simulink model "fuzzy_AG"  (R2022b)
settings: Solver=VariableStepAuto  StartTime=0.0  StopTime=20000  RelTol=1e-3
libraries: fuzblock x1
settings Model: Creator=Juan Jose Restrepo  LastModifiedBy=mluser

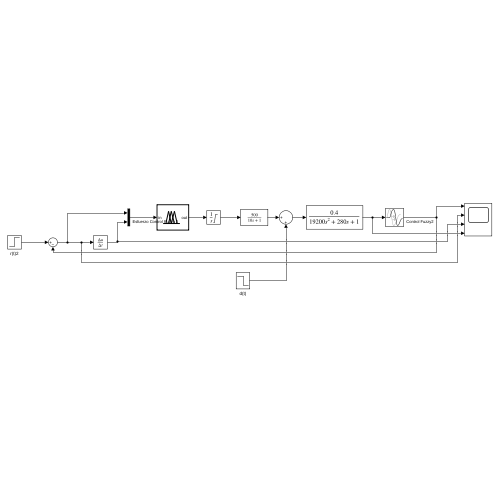
[thumbnail: Simulink's stored preview of the top-level diagram]
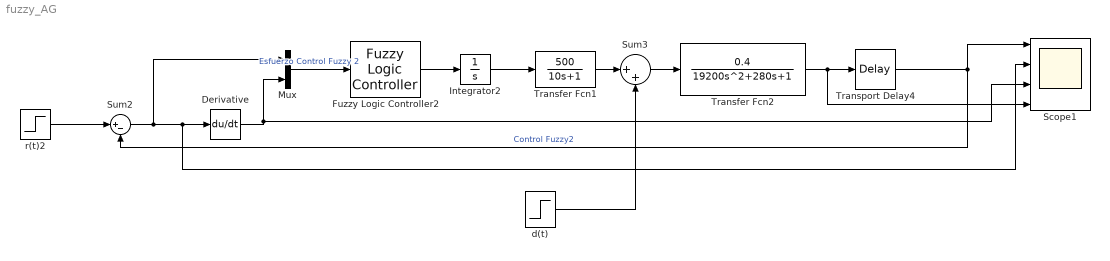
== system fuzzy_AG ==
  Derivative : Derivative
  Fuzzy Logic Controller2 : fuzblock/Fuzzy Logic  Controller  FIS=V6_fuzzyMarco  OutputSampleNumber=101  DataType=double  FuzzifiedInputs=off  RuleFiringStrengths=off  RuleOutputs=off  AggregatedOutputs=off  SimulateUsing=Interpreted execution  OutOfRangeInputValueMessage=warning  NoRuleFiredMessage=warning  EmptyOutputFuzzySetMessage=warning
  Integrator2 : Integrator  LimitOutput=on  UpperSaturationLimit=0.02  LowerSaturationLimit=0
  Mux : Mux  Inputs=2
  Scope1 : Scope  NumInputPorts=4
  Sum2 : Sum  Inputs=|+-
  Sum3 : Sum  Inputs=|++
  Transfer Fcn1 : TransferFcn  Numerator=[500]  Denominator=[10 1]
  Transfer Fcn2 : TransferFcn  Numerator=[0.4]  Denominator=[19200 280 1]
  Transport Delay4 : TransportDelay  DelayTime=120
  d(t) : Step  Time=10000  After=-1  SampleTime=0
  r(t)2 : Step  Time=0  After=1.5  SampleTime=0
  wires:
  Transfer Fcn1/1 -> Sum3/1
  Transfer Fcn2/1 -> Scope1/4, Transport Delay4/1
  Integrator2/1 -> Transfer Fcn1/1
  Sum3/1 -> Transfer Fcn2/1
  Fuzzy Logic Controller2/1 -> Integrator2/1
  r(t)2/1 -> Sum2/1
  Derivative/1 -> Mux/2, Scope1/3
  Mux/1 -> Fuzzy Logic Controller2/1  "Esfuerzo Control Fuzzy 2"
  Sum2/1 -> Mux/1, Scope1/2, Derivative/1
  Transport Delay4/1 -> Scope1/1, Sum2/2  "Control Fuzzy2"
  d(t)/1 -> Sum3/2
